simulink model "model_tmp_4p"  (R2015b)
settings: Solver=ode45  StartTime=0.0  StopTime=T_sim  FixedStep=dt  RelTol=1e-3
PreLoadFcn:
  | setup_tmp_4p;
InitFcn:
  | setup_tmp_4p;
StartFcn:
  | setup_tmp_4p;
values from neighbouring files (symbols this model uses):
  A_act = [-100 0 0 0 0 -100 0 0 0 0 -100 0 ... (16 elements, 4x4)]    [CD_spline.mat]    (also in CL_spline.mat; setup.m = -100*eye(4); setup_tmp_1p.m = -100*eye(4); setup_tmp_4p.m = -100*eye(4))
  A_init = [1.0386 0 12.9]    [CD_spline.mat]    (also in CL_spline.mat; setup_KiteModel_4points.m = Pc_init + d_n_r * w_k * w_rel * [-1;0;0])
  A_Kite = 7    [CD_spline.mat]    (also in CL_spline.mat; setup.m = 10.18; setup_tmp_1p.m = 10.18; setup_tmp_4p.m = 10.18)
  A_prd = [0 0 0 -640 0 0 0 0 0 0 -640 0 ... (36 elements, 6x6)]    [CD_spline.mat]    (also in CL_spline.mat; setup.m = 1000 * A_M_aug; setup_tmp_1p.m = 1000 * A_M_aug; setup_tmp_4p.m = 1000 * A_M_aug)
  A_ref = [0 0 0 -10000 0 0 0 0 0 0 -10000 0 ... (36 elements, 6x6)]    [CD_spline.mat]    (also in CL_spline.mat; setup.m = zeros(6); setup_tmp_1p.m = zeros(6); setup_tmp_4p.m = zeros(6))
  A_t_ref_cl = [0 0 0 -0.64 0 0 0 0 0 0 -0.64 0 ... (36 elements, 6x6)]    [CD_spline.mat]    (also in CL_spline.mat; setup.m = A_t_ref; setup_tmp_1p.m = A_t_ref; setup_tmp_4p.m = A_t_ref)
  alpha_0 = 10 * pi/180    (= 0.174532925199)    [setup_KiteModel_4points.m]
  alpha_d_max = 31 * pi/180    (= 0.541052068118)    [setup_KiteModel_4points.m]
  alpha_s_0 = 10 * pi/180    (= 0.174532925199)    [setup_KiteModel_4points.m]
  alpha_s_max = 20 * pi/180    (= 0.349065850399)    [setup_KiteModel_4points.m]
  ASideRel = 0    [CD_spline.mat]    (also in CL_spline.mat; setup.m; setup_tmp_1p.m; setup_tmp_4p.m = 0.306)
  B_act = [100 0 0 0 0 100 0 0 0 0 100 0 ... (16 elements, 4x4)]    [CD_spline.mat]    (also in CL_spline.mat; setup.m = 100*eye(4); setup_tmp_1p.m = 100*eye(4); setup_tmp_4p.m = 100*eye(4))
  B_init = [0 0 15.13]    [CD_spline.mat]    (also in CL_spline.mat; setup_KiteModel_4points.m = Pc_init + h_kite * [0;0;1;])
  B_ref = [0 0 0 10000 0 0 0 0 0 0 10000 0 ... (18 elements, 6x3)]    [CD_spline.mat]    (also in CL_spline.mat; setup.m = zeros(6,3); setup_tmp_1p.m = zeros(6,3); setup_tmp_4p.m = zeros(6,3))
  B_t_ref_cl = [0 0 0 0.64 0 0 0 0 0 0 0.64 0 ... (18 elements, 6x3)]    [CD_spline.mat]    (also in CL_spline.mat)
  Bpbl = [0 0 0 1 0 0 0 0 0 0 1 0 ... (18 elements, 6x3)]    [CD_spline.mat]    (also in CL_spline.mat; setup.m = [zeros(3); eye(3)]; setup_tmp_1p.m = [zeros(3); eye(3)]; setup_tmp_4p.m = [zeros(3); eye(3)])
  c0 = 614000    [CD_spline.mat]    (also in CL_spline.mat; setup.m; setup_tmp_1p.m; setup_tmp_4p.m)
  c_1_TR = 0.262    [setup_KiteModel_4points.m]
  C_A = [0 0.3 -1e-06 1 -0.3 0 1e-06 1 0 -0.3 -1e-06 1 ... (16 elements, 4x4)]    [CD_spline.mat]    (also in CL_spline.mat; setup.m = [0, -R, 0, R; setup_tmp_1p.m = [0, -R, 0, R; setup_tmp_4p.m = [0, -R, 0, R)
  C_A_inv = [0 -1.66666666667 -1.23358113847e-17 1.66666666667 1.66666666667 2.46716227694e-17 -1.66666666667 0 -250000 250000 -250000 250000 ... (16 elements, 4x4)]    [CD_spline.mat]    (also in CL_spline.mat; setup.m = C_A \eye(4); setup_tmp_1p.m = C_A \eye(4); setup_tmp_4p.m = C_A \eye(4))
  C_init = [0 2.5965 12.9]    [CD_spline.mat]    (also in CL_spline.mat; setup_KiteModel_4points.m = Pc_init + 0.5 * w_k * w_rel * [0;1;0])
  CD_spline_coefs = CD_spline.coefs    [setup_KiteModel_4points.m]
  CD_tether = 0.96    [CD_spline.mat]    (also in CL_spline.mat; setup.m; setup_tmp_1p.m; setup_tmp_4p.m)
  CL_spline_coefs = CL_spline.coefs    [setup_KiteModel_4points.m]
  d0 = 473    [CD_spline.mat]    (also in CL_spline.mat; setup.m; setup_tmp_1p.m; setup_tmp_4p.m)
  D_init = [0 -2.5965 12.9]    [CD_spline.mat]    (also in CL_spline.mat; setup_KiteModel_4points.m = Pc_init - 0.5 * w_k * w_rel * [0;1;0])
  d_tether = 0.004    [CD_spline.mat]    (also in CL_spline.mat; setup.m; setup_tmp_1p.m; setup_tmp_4p.m)
  delta_dead = 0.5    [CD_spline.mat]    (also in CL_spline.mat; setup.m; setup_tmp_1p.m; setup_tmp_4p.m)
  e_0 = 0.01    [CD_spline.mat]    (also in CL_spline.mat; setup.m; setup_tmp_1p.m; setup_tmp_4p.m)
  epsilon = 0.6    [CD_spline.mat]    (also in CL_spline.mat; setup.m; setup_tmp_1p.m; setup_tmp_4p.m)
  g = 9.81    [CD_spline.mat]    (also in CL_spline.mat; setup.m; setup_tmp_1p.m; setup_tmp_4p.m)
  g_vec = [0 0 9.81]    [CD_spline.mat]    (also in CL_spline.mat; setup.m = [0;0;9.81]; setup_tmp_1p.m = [0;0;9.81]; setup_tmp_4p.m = [0;0;9.81])
  Gamma_ad = 100    [CD_spline.mat]    (also in CL_spline.mat; setup.m = 100;100; setup_tmp_1p.m = 100;100; setup_tmp_4p.m = 100;100)
  Gamma_pred = 100    [CD_spline.mat]    (also in CL_spline.mat; setup.m; setup_tmp_1p.m; setup_tmp_4p.m)
  J = [0.018  0  0; 0  0.018  0; 0  0  0.009]    [CD_spline.mat]    (also in CL_spline.mat; setup.m = diag([Ixx, Iyy, Izz]); setup_tmp_1p.m = diag([Ixx, Iyy, Izz]); setup_tmp_4p.m = diag([Ixx, Iyy, Izz]))
  Jinv = [55.5555555556  0  0; 0  55.5555555556  0; 0  0  111.111111111]    [CD_spline.mat]    (also in CL_spline.mat; setup.m = J \ eye(3); setup_tmp_1p.m = J \ eye(3); setup_tmp_4p.m = J \ eye(3))
  K = 1 - ASideRel    [setup_KiteModel_4points.m]
  K_d_s = 1.5    [setup_KiteModel_4points.m]
  k_e_eta = 10000    [CD_spline.mat]    (also in CL_spline.mat; setup.m; setup_tmp_1p.m; setup_tmp_4p.m)
  k_e_eta_dot = 400    [CD_spline.mat]    (also in CL_spline.mat; setup.m; setup_tmp_1p.m; setup_tmp_4p.m)
  k_e_eta_I = 1    [CD_spline.mat]    (also in CL_spline.mat; setup.m; setup_tmp_1p.m; setup_tmp_4p.m)
  K_e_psi = 10    [setup_tmp_4p.m]
  K_i_t = [10  0  0; 0  10  0; 0  0  10]    [CD_spline.mat]    (also in CL_spline.mat; setup.m = 10*eye(3); setup_tmp_1p.m = 10*eye(3); setup_tmp_4p.m = 10*eye(3))
  K_v_t = [1.6  0  0; 0  1.6  0; 0  0  1.6]    [CD_spline.mat]    (also in CL_spline.mat; setup.m = 2*omega_0_trans*zeta_0_trans*eye(3); setup_tmp_1p.m = 2*omega_0_trans*zeta_0_trans*eye(3); setup_tmp_4p.m = 2*omega_0_trans*zeta_0_trans*eye(3))
  K_x_t = [0.64  0  0; 0  0.64  0; 0  0  0.64]    [CD_spline.mat]    (also in CL_spline.mat; setup.m = omega_0_trans^2*eye(3); setup_tmp_1p.m = omega_0_trans^2*eye(3); setup_tmp_4p.m = omega_0_trans^2*eye(3))
  l_s0 = 1    [CD_spline.mat]    (also in CL_spline.mat; setup.m = 1.42857142857; setup_tmp_1p.m = 1.42857142857; setup_tmp_4p.m = 2)
  l_s_BP = norm( B_init - p_B_UAV_init)    [setup_KiteModel_4points.m]
  l_s_PUav = norm( pos_UAV_init - p_B_UAV_init)    [setup_KiteModel_4points.m]
  ls_AB = norm( A_init -  B_init)    [setup_KiteModel_4points.m]
  ls_AC = norm( A_init -  C_init)    [setup_KiteModel_4points.m]
  ls_AD = norm( A_init -  D_init)    [setup_KiteModel_4points.m]
  ls_AKcu = norm( A_init -  P_kcu)    [setup_KiteModel_4points.m]
  ls_CB = norm( C_init -  B_init)    [setup_KiteModel_4points.m]
  ls_CD = norm( C_init -  D_init)    [setup_KiteModel_4points.m]
  ls_CKcu = norm( C_init - P_kcu)    [setup_KiteModel_4points.m]
  ls_DB = norm( D_init - B_init )    [setup_KiteModel_4points.m]
  ls_DKcu = norm( D_init - P_kcu)    [setup_KiteModel_4points.m]
  m_A = 3.29    [CD_spline.mat]    (also in CL_spline.mat; setup_KiteModel_4points.m = nose_mass_fraction * m_kite)
  m_B = 1.484    [CD_spline.mat]    (also in CL_spline.mat; setup_KiteModel_4points.m = 0.4 * (1-nose_mass_fraction)*m_kite)
  m_C = 1.113    [CD_spline.mat]    (also in CL_spline.mat; setup_KiteModel_4points.m = 0.3 * (1-nose_mass_fraction)*m_kite)
  m_D = 1.113    [CD_spline.mat]    (also in CL_spline.mat; setup_KiteModel_4points.m = 0.3 * (1-nose_mass_fraction)*m_kite)
  m_kcu = 8.4    [setup_tmp_4p.m]
  m_p = 0.013    [CD_spline.mat]    (also in CL_spline.mat; setup.m = 0.0185714285714; setup_tmp_1p.m = 0.0185714285714; setup_tmp_4p.m = 0.026)
  m_uav = 3    [CD_spline.mat]    (also in CL_spline.mat; setup.m; setup_tmp_1p.m; setup_tmp_4p.m)
  n_t_p = 7    [setup.m]    (also in setup_tmp_1p.m; setup_tmp_4p.m = 5)
  p_B_UAV_init = B_init + [0;0;l_s0]    [setup_KiteModel_4points.m]
  p_init_4p = zeros(3*n_t_p,1)    [setup.m]    (also in setup_tmp_4p.m)
  P_prd = [712.5 0 0 156.25 0 0 0 712.5 0 0 156.25 0 ... (36 elements, 6x6)]    [CD_spline.mat]    (also in CL_spline.mat; setup.m = 1000 * P_tref; setup_tmp_1p.m = 1000 * P_tref; setup_tmp_4p.m = 1000 * P_tref)
  P_tref = [0.7125 0 0 0.15625 0 0 0 0.7125 0 0 0.15625 0 ... (36 elements, 6x6)]    [CD_spline.mat]    (also in CL_spline.mat; setup.m = lyap(A_M_aug', Q); setup_tmp_1p.m = lyap(A_M_aug', Q); setup_tmp_4p.m = lyap(A_M_aug', Q))
  pos_UAV_init = p_B_UAV_init + [0;0;l_s0]    [setup_KiteModel_4points.m]
  rho_air = 1.225    [CD_spline.mat]    (also in CL_spline.mat; setup.m; setup_tmp_1p.m; setup_tmp_4p.m)
  rho_t = 0.013    [CD_spline.mat]    (also in CL_spline.mat; setup.m; setup_tmp_1p.m; setup_tmp_4p.m)
  sample_log = 0.01    [CD_spline.mat]    (also in CL_spline.mat; setup.m; setup_tmp_1p.m; setup_tmp_4p.m)
  T_launch = 40    [CD_spline.mat]    (also in CL_spline.mat; setup.m; setup_tmp_1p.m; setup_tmp_4p.m)
  Theta_max = 60    [CD_spline.mat]    (also in CL_spline.mat; setup.m; setup_tmp_1p.m; setup_tmp_4p.m)
  Thrust_Max = 80    [CD_spline.mat]    (also in CL_spline.mat; setup.m; setup_tmp_1p.m = 100; setup_tmp_4p.m = 1000000000)
  Tx = 10    [CD_spline.mat]    (also in CL_spline.mat; setup.m; setup_tmp_1p.m; setup_tmp_4p.m)
  Ty = 10    [CD_spline.mat]    (also in CL_spline.mat; setup.m; setup_tmp_1p.m; setup_tmp_4p.m)
  Tz = 10    [CD_spline.mat]    (also in CL_spline.mat; setup.m; setup_tmp_1p.m; setup_tmp_4p.m)
  u_d_0 = 0.213    [setup_KiteModel_4points.m]
  u_d_max = 0.47    [setup_KiteModel_4points.m]
  u_s_0 = 0    [setup_KiteModel_4points.m]
  v_w_vec = [1 1 1]    [CD_spline.mat]    (also in CL_spline.mat; setup.m = [1;0;0]; setup_tmp_1p.m = [1;0;0]; setup_tmp_4p.m = [0.01;0;0])
  x0num = 0    [CD_spline.mat]    (also in CL_spline.mat; polynomial_trajectory.m = double( solutions_x.x0 ))
  x1num = 0    [CD_spline.mat]    (also in CL_spline.mat; polynomial_trajectory.m = double( solutions_x.x1 ))
  x2num = 0    [CD_spline.mat]    (also in CL_spline.mat; polynomial_trajectory.m = double( solutions_x.x2 ))
  x3num = 0.05    [CD_spline.mat]    (also in CL_spline.mat; polynomial_trajectory.m = double( solutions_x.x3 ))
  x4num = -0.0075    [CD_spline.mat]    (also in CL_spline.mat; polynomial_trajectory.m = double( solutions_x.x4 ))
  x5num = 0.0003    [CD_spline.mat]    (also in CL_spline.mat; polynomial_trajectory.m = double( solutions_x.x5 ))
  x_drone_init = [0 0 10]    [CD_spline.mat]    (also in CL_spline.mat; setup.m = p_init(3*n-2:3*n); setup_KiteModel_4points.m = pos_UAV_init; setup_tmp_1p.m = p_init(3*n-2:3*n))
  xT = 5    [CD_spline.mat]    (also in CL_spline.mat; setup.m; setup_tmp_1p.m = 10; setup_tmp_4p.m = 10)
  y0num = 0    [CD_spline.mat]    (also in CL_spline.mat; polynomial_trajectory.m = double( solutions_y.y0 ))
  y1num = 0    [CD_spline.mat]    (also in CL_spline.mat; polynomial_trajectory.m = double( solutions_y.y1 ))
  y2num = 0    [CD_spline.mat]    (also in CL_spline.mat; polynomial_trajectory.m = double( solutions_y.y2 ))
  y3num = 0.1    [CD_spline.mat]    (also in CL_spline.mat; polynomial_trajectory.m = double( solutions_y.y3 ))
  y4num = -0.015    [CD_spline.mat]    (also in CL_spline.mat; polynomial_trajectory.m = double( solutions_y.y4 ))
  y5num = 0.0006    [CD_spline.mat]    (also in CL_spline.mat; polynomial_trajectory.m = double( solutions_y.y5 ))
  yT = 10    [CD_spline.mat]    (also in CL_spline.mat; setup.m; setup_tmp_1p.m = 0; setup_tmp_4p.m = 0)
  z0num = 10    [CD_spline.mat]    (also in CL_spline.mat; polynomial_trajectory.m = double( solutions_z.z0 ))
  z1num = 0    [CD_spline.mat]    (also in CL_spline.mat; polynomial_trajectory.m = double( solutions_z.z1 ))
  z2num = 0    [CD_spline.mat]    (also in CL_spline.mat; polynomial_trajectory.m = double( solutions_z.z2 ))
  z3num = 0.4    [CD_spline.mat]    (also in CL_spline.mat; polynomial_trajectory.m = double( solutions_z.z3 ))
  z4num = -0.06    [CD_spline.mat]    (also in CL_spline.mat; polynomial_trajectory.m = double( solutions_z.z4 ))
  z5num = 0.0024    [CD_spline.mat]    (also in CL_spline.mat; polynomial_trajectory.m = double( solutions_z.z5 ))
  zT = 50    [CD_spline.mat]    (also in CL_spline.mat; setup.m; setup_tmp_1p.m; setup_tmp_4p.m)
libraries: simulink x1
(part 2 of 3)

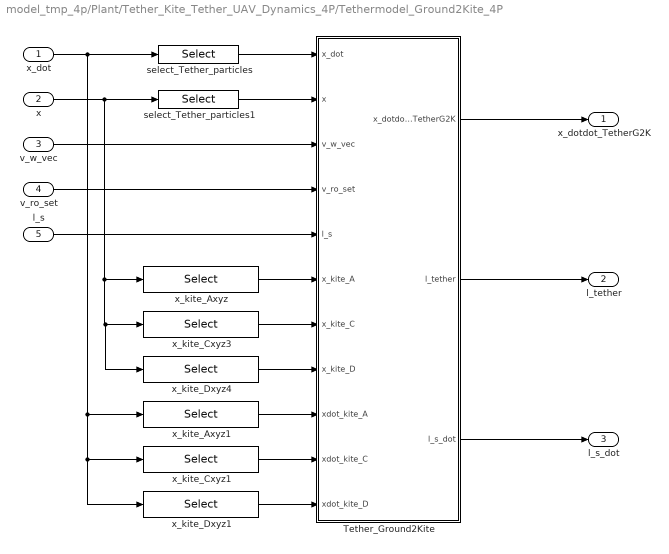
== system model_tmp_4p/Plant/Tether_Kite_Tether_UAV_Dynamics_4P/Tethermodel_Ground2Kite_4P ==
  x_dot : Inport
  x : Inport  Port=2
  v_w_vec : Inport  Port=3
  v_ro_set : Inport  Port=4
  l_s : Inport  Port=5
  Tether_Ground2Kite : MATLAB Function  TreatAsAtomicUnit=on
  select_Tether_particles : Selector  InputPortWidth=3*n_t_p+18  IndexOptions=Index vector (dialog)  Indices=[1 : 3*n_t_p]  OutputSizes=1
  select_Tether_particles1 : Selector  InputPortWidth=3*n_t_p+18  IndexOptions=Index vector (dialog)  Indices=[1 : 3*n_t_p]  OutputSizes=1
  x_kite_Axyz : Selector  InputPortWidth=3*n_t_p+18  IndexOptions=Index vector (dialog)  Indices=[3*n_t_p+1:3*n_t_p+3]  OutputSizes=1
  x_kite_Axyz1 : Selector  InputPortWidth=3*n_t_p+18  IndexOptions=Index vector (dialog)  Indices=[3*n_t_p+1:3*n_t_p+3]  OutputSizes=1
  x_kite_Cxyz1 : Selector  InputPortWidth=3*n_t_p+18  IndexOptions=Index vector (dialog)  Indices=[3*n_t_p+7:3*n_t_p+9]  OutputSizes=1
  x_kite_Cxyz3 : Selector  InputPortWidth=3*n_t_p+18  IndexOptions=Index vector (dialog)  Indices=[3*n_t_p+7:3*n_t_p+9]  OutputSizes=1
  x_kite_Dxyz1 : Selector  InputPortWidth=3*n_t_p+18  IndexOptions=Index vector (dialog)  Indices=[3*n_t_p+10:3*n_t_p+12]  OutputSizes=1
  x_kite_Dxyz4 : Selector  InputPortWidth=3*n_t_p+18  IndexOptions=Index vector (dialog)  Indices=[3*n_t_p+10:3*n_t_p+12]  OutputSizes=1
  x_dotdot_TetherG2K : Outport
  l_tether : Outport  Port=2
  l_s_dot : Outport  Port=3
  wires:
  v_w_vec/1 -> Tether_Ground2Kite/3(v_w_vec)
  x_dot/1 -> x_kite_Dxyz1/1, x_kite_Cxyz1/1, x_kite_Axyz1/1, select_Tether_particles/1
  x/1 -> x_kite_Dxyz4/1, x_kite_Cxyz3/1, x_kite_Axyz/1, select_Tether_particles1/1
  Tether_Ground2Kite/1(x_dotdot_TetherG2K) -> x_dotdot_TetherG2K/1
  Tether_Ground2Kite/2(l_tether) -> l_tether/1
  Tether_Ground2Kite/3(l_s_dot) -> l_s_dot/1
  l_s/1 -> Tether_Ground2Kite/5(l_s)
  v_ro_set/1 -> Tether_Ground2Kite/4(v_ro_set)
  select_Tether_particles/1 -> Tether_Ground2Kite/1(x_dot)
  select_Tether_particles1/1 -> Tether_Ground2Kite/2(x)
  x_kite_Axyz/1 -> Tether_Ground2Kite/6(x_kite_A)
  x_kite_Cxyz3/1 -> Tether_Ground2Kite/7(x_kite_C)
  x_kite_Dxyz4/1 -> Tether_Ground2Kite/8(x_kite_D)
  x_kite_Axyz1/1 -> Tether_Ground2Kite/9(xdot_kite_A)
  x_kite_Dxyz1/1 -> Tether_Ground2Kite/11(xdot_kite_D)
  x_kite_Cxyz1/1 -> Tether_Ground2Kite/10(xdot_kite_C)

== system model_tmp_4p/Plant/Tether_Kite_Tether_UAV_Dynamics_4P/Tethermodel_Kite2UAV ==
  x_p_dot : Inport
  launch_flag : Inport  Port=2
  x_p : Inport  Port=3
  v_w_vec : Inport  Port=4
  Tether_Kite2UAV : MATLAB Function  TreatAsAtomicUnit=on
  particle between uav and kite : Selector  InputPortWidth=3*n_t_p +18  IndexOptions=Index vector (dialog)  Indices=[3*n_t_p+13: 3*n_t_p+15]  OutputSizes=1
  particle between uav and kite1 : Selector  InputPortWidth=3*n_t_p +18  IndexOptions=Index vector (dialog)  Indices=[3*n_t_p+13: 3*n_t_p+15]  OutputSizes=1
  uav : Selector  InputPortWidth=3*n_t_p +18  IndexOptions=Index vector (dialog)  Indices=[3*n_t_p + 16: 3*n_t_p + 18]  OutputSizes=1
  x_kite_B : Selector  InputPortWidth=3*n_t_p +18  IndexOptions=Index vector (dialog)  Indices=[3*n_t_p + 4: 3*n_t_p + 6]  OutputSizes=1
  x_kite_B1 : Selector  InputPortWidth=3*n_t_p +18  IndexOptions=Index vector (dialog)  Indices=[3*n_t_p + 4: 3*n_t_p + 6]  OutputSizes=1
  x_kite_B5 : Selector  InputPortWidth=3*n_t_p +18  IndexOptions=Index vector (dialog)  Indices=[3*n_t_p + 16: 3*n_t_p + 18]  OutputSizes=1
  x_dotdot_p : Outport
  wires:
  Tether_Kite2UAV/1(x_dotdot_p) -> x_dotdot_p/1
  launch_flag/1 -> Tether_Kite2UAV/1(launch_flag)
  uav/1 -> Tether_Kite2UAV/2(xp_above)
  x_kite_B1/1 -> Tether_Kite2UAV/7(xp_dot_below)
  x_p_dot/1 -> particle between uav and kite1/1, x_kite_B1/1, x_kite_B5/1
  particle between uav and kite/1 -> Tether_Kite2UAV/3(xp)
  x_kite_B5/1 -> Tether_Kite2UAV/5(xp_dot_above)
  x_p/1 -> uav/1, particle between uav and kite/1, x_kite_B/1
  x_kite_B/1 -> Tether_Kite2UAV/4(xp_below)
  v_w_vec/1 -> Tether_Kite2UAV/8(v_w_vec)
  particle between uav and kite1/1 -> Tether_Kite2UAV/6(xp_dot)

== system model_tmp_4p/Plant/Tether_Kite_Tether_UAV_Dynamics_4P/UAV_Model ==
  x_p_dot : Inport
  x_p : Inport  Port=2
  u_M : Inport  Port=3
  u_Thrust_I : Inport  Port=4
  eta : Inport  Port=5
  omega : Inport  Port=6
  Kite1 : Selector  InputPortWidth=3*n_t_p + 18  IndexOptions=Index vector (dialog)  Indices=[3*n_t_p + 16:3*n_t_p + 18]  OutputSizes=1
  Kite2 : Selector  InputPortWidth=3*n_t_p + 18  IndexOptions=Index vector (dialog)  Indices=[3*n_t_p + 16:3*n_t_p + 18]  OutputSizes=1
  Kite3 : Selector  InputPortWidth=3*n_t_p + 18  IndexOptions=Index vector (dialog)  Indices=[3*n_t_p + 13:3*n_t_p + 15]  OutputSizes=1
  Kite4 : Selector  InputPortWidth=3*n_t_p + 18  IndexOptions=Index vector (dialog)  Indices=[3*n_t_p + 13:3*n_t_p + 15]  OutputSizes=1
  Rotate thrust vector according to attitude : MATLAB Function  TreatAsAtomicUnit=on
  To Workspace4 : ToWorkspace  VariableName=F_T_b  SaveFormat=Timeseries  SampleTime=sample_log
  UAV_Dynamics : MATLAB Function  TreatAsAtomicUnit=on
  x_dotdot_uav : Outport
  omega_dot : Outport  Port=2
  eta_dot : Outport  Port=3
  tag scope: disturbance=global
  wires:
  Rotate thrust vector according to attitude/1(u_Thrust_B) -> To Workspace4/1, UAV_Dynamics/1(Thrust)
  UAV_Dynamics/1(x_dotdot_uav_trans) -> x_dotdot_uav/1
  Kite1/1 -> UAV_Dynamics/2(x_UAV)
  Kite4/1 -> UAV_Dynamics/5(x_dot_belowUAV)
  Kite2/1 -> UAV_Dynamics/4(x_dot_UAV)
  x_p_dot/1 -> Kite4/1, Kite2/1
  x_p/1 -> Kite3/1, Kite1/1
  UAV_Dynamics/4(disturbance) -> [disturbance]
  UAV_Dynamics/2(omega_dot) -> omega_dot/1
  UAV_Dynamics/3(eta_dot) -> eta_dot/1
  u_M/1 -> UAV_Dynamics/7(u_M)
  eta/1 -> Rotate thrust vector according to attitude/2(eta), UAV_Dynamics/8(eta)
  omega/1 -> UAV_Dynamics/6(omega)
  u_Thrust_I/1 -> Rotate thrust vector according to attitude/1(u_Thrust_I)
  Kite3/1 -> UAV_Dynamics/3(x_below_UAV)

== system model_tmp_4p/Controller/Outer_Loop_Position/Adaptive_Augmentation/Proj(Theta_hat, GammaY)_1column ==
  note: Ref.: Lavretsky, Robust and Adaptive Control, p. 329
      | Lecure Notes Nonlinear and Adaptive Control, TU Munich, FSD, SS2014, Robustness Modifications
  Theta_hat : Inport
  Theta_dot : Inport  Port=2
  Mux : Mux  Inputs=3
  Proj(Theta,Theta_dot) : MATLAB Function  TreatAsAtomicUnit=on
  Reshape1 : Reshape  OutputDimensionality=Row vector (2-D)
  Reshape2 : Reshape  OutputDimensionality=Row vector (2-D)
  To Workspace1 : ToWorkspace  VariableName=proj_flat  SaveFormat=Timeseries  SampleTime=sample_log
      settings: Save2DSignal=2-D array (concatenate along first dimension)
  To Workspace2 : ToWorkspace  VariableName=Theta_dot_save  SampleTime=sample_log
      settings: Save2DSignal=2-D array (concatenate along first dimension)
  To Workspace3 : ToWorkspace  VariableName=orthogonal_part  SampleTime=sample_log
      settings: Save2DSignal=2-D array (concatenate along first dimension)
  calculate_f : MATLAB Function  TreatAsAtomicUnit=on
  calculate_gradf : MATLAB Function  TreatAsAtomicUnit=on
  max_allowable_bound : Constant  Value=Theta_max
  projection_tolerance : Constant  Value=epsilon
  Theta_hat_dot : Outport
  wires:
  Proj(Theta,Theta_dot)/2(Theta_hat_dot_) -> Reshape1/1, Theta_hat_dot/1
  Proj(Theta,Theta_dot)/1(flag) -> Mux/2
  Proj(Theta,Theta_dot)/3(direction) -> Mux/3
  Mux/1 -> To Workspace1/1
  calculate_gradf/1(gradf) -> Proj(Theta,Theta_dot)/2(gradf)
  Theta_hat/1 -> calculate_gradf/1(theta_hat), calculate_f/1(theta_hat)
  projection_tolerance/1 -> calculate_f/3(epsilon), calculate_gradf/3(epsilon)
  max_allowable_bound/1 -> calculate_f/2(Theta_max), calculate_gradf/2(Theta_max)
  Theta_dot/1 -> Proj(Theta,Theta_dot)/3(Theta_dot)
  calculate_f/1(f) -> Mux/1, Proj(Theta,Theta_dot)/1(f)
  Reshape1/1 -> To Workspace2/1
  Proj(Theta,Theta_dot)/4(orthogonal_part) -> Reshape2/1
  Reshape2/1 -> To Workspace3/1

== system model_tmp_4p/Controller/Outer_Loop_Position/Adaptive_Augmentation/Proj(Theta_hat, GammaY)_multicolumns ==
  note: Ref.: Lavretsky, Robust and Adaptive Control, p. 329
      | Lecure Notes Nonlinear and Adaptive Control, TU Munich, FSD, SS2014, Robustness Modifications
  Theta_hat : Inport
  Theta_dot : Inport  Port=2
  MATLAB Function : MATLAB Function  TreatAsAtomicUnit=on
  Matrix Concatenate : Concatenate  NumInputs=3  Mode=Multidimensional array
  Projection_Input_1 : Subsystem
  Projection_Input_2 : Subsystem
  Projection_Input_3 : Subsystem
  Theta_hat_dot : Outport
  wires:
  Theta_hat/1 -> MATLAB Function/1(Theta_hat)
  Theta_dot/1 -> MATLAB Function/2(Theta_hat_dot)
  Projection_Input_1/1(Out1) -> Matrix Concatenate/1
  MATLAB Function/1(Theta_hat_1) -> Projection_Input_1/1(In1)
  MATLAB Function/2(Theta_hat_dot_1) -> Projection_Input_1/2(In2)
  MATLAB Function/3(Theta_hat_2) -> Projection_Input_2/1(In1)
  MATLAB Function/4(Theta_hat_dot_2) -> Projection_Input_2/2(In2)
  MATLAB Function/6(Theta_hat_dot_3) -> Projection_Input_3/2(In2)
  MATLAB Function/5(Theta_hat_3) -> Projection_Input_3/1(In1)
  Projection_Input_2/1(Out1) -> Matrix Concatenate/2
  Projection_Input_3/1(Out1) -> Matrix Concatenate/3
  Matrix Concatenate/1 -> Theta_hat_dot/1

== system model_tmp_4p/Controller/Outer_Loop_Position/Adaptive_Augmentation/Smooth_Deadzone_MRAC ==
  note: Ref.: Lavretsky, Robust and Adaptive Control, p. 319
  e : Inport
  Dead_Zone_Mod1 : Constant  Value=delta_dead
  Dead_Zone_Mod2 : Constant  Value=e_0
  Dot Product : DotProduct  InputSameDT=on  OutDataTypeStr=Inherit: Inherit via internal rule
  Mux : Mux  Inputs=2
  Sqrt : Sqrt  SaturateOnIntegerOverflow=on
  To Workspace8 : ToWorkspace  VariableName=e_ref_mu  SaveFormat=Timeseries  SampleTime=sample_log
      settings: Save2DSignal=2-D array (concatenate along first dimension)
  smooth_deadzone : MATLAB Function  TreatAsAtomicUnit=on
  mu_dead : Outport
  wires:
  e/1 -> Dot Product/1, Dot Product/2
  Dead_Zone_Mod1/1 -> smooth_deadzone/2(delta_dead)
  Dead_Zone_Mod2/1 -> smooth_deadzone/3(e_0)
  Dot Product/1 -> Sqrt/1
  Sqrt/1 -> Mux/1, smooth_deadzone/1(e_norm)
  smooth_deadzone/1(mu_dead) -> Mux/2, mu_dead/1
  Mux/1 -> To Workspace8/1

== system model_tmp_4p/Controller/Outer_Loop_Position/Adaptive_Augmentation/Smooth_Deadzone_PMRAC ==
  note: Ref.: Lavretsky, Robust and Adaptive Control, p. 319
  e : Inport
  Dead_Zone_Mod1 : Constant  Value=delta_dead
  Dead_Zone_Mod2 : Constant  Value=e_0
  Dot Product : DotProduct  InputSameDT=on  OutDataTypeStr=Inherit: Inherit via internal rule
  Mux1 : Mux  Inputs=2
  Sqrt : Sqrt  SaturateOnIntegerOverflow=on
  To Workspace1 : ToWorkspace  VariableName=e_pref_mu  SaveFormat=Timeseries  SampleTime=sample_log
      settings: Save2DSignal=2-D array (concatenate along first dimension)
  smooth_deadzone : MATLAB Function  TreatAsAtomicUnit=on
  mu_dead : Outport
  wires:
  Dot Product/1 -> Sqrt/1
  Dead_Zone_Mod2/1 -> smooth_deadzone/3(e_0)
  Dead_Zone_Mod1/1 -> smooth_deadzone/2(delta_dead)
  e/1 -> Dot Product/2, Dot Product/1
  Sqrt/1 -> Mux1/1, smooth_deadzone/1(e_norm)
  smooth_deadzone/1(mu_dead) -> Mux1/2, mu_dead/1
  Mux1/1 -> To Workspace1/1

== system model_tmp_4p/Plant/Tether_Kite_Tether_UAV_Dynamics_4P/First_order_lag_Actuator/Actuator ==
  Propeller_RPMs_cmd : Inport
  Add : Sum  Inputs=+-
  Gain : Gain  Gain=B_act  Multiplication=Matrix(K*u)
  Gain1 : Gain  Gain=A_act  Multiplication=Matrix(K*u)
  Integrator Limited1 : Integrator  InitialCondition=zeros(4,1)  LimitOutput=on  UpperSaturationLimit=Thrust_Max  LowerSaturationLimit=-Thrust_Max
  Output_Actuator : Gain  Gain=C_A  Multiplication=Matrix(K*u)
  Reaction_Deficit_Actuators : Scope
  Sum : Sum  Inputs=|++
  To Workspace1 : ToWorkspace  VariableName=prop_thrust_cmd  SaveFormat=Timeseries  SampleTime=sample_log
  To Workspace2 : ToWorkspace  VariableName=prop_thrust_real  SaveFormat=Timeseries  SampleTime=sample_log
  Thrust_Moments : Outport
  wires:
  Output_Actuator/1 -> Thrust_Moments/1
  Gain/1 -> Sum/1
  Gain1/1 -> Sum/2
  Sum/1 -> Integrator Limited1/1
  Propeller_RPMs_cmd/1 -> Add/1, To Workspace1/1, Gain/1
  Add/1 -> Reaction_Deficit_Actuators/1
  Integrator Limited1/1 -> Add/2, To Workspace2/1, Gain1/1, Output_Actuator/1

== system model_tmp_4p/Controller/Outer_Loop_Position/Adaptive_Augmentation/Proj(Theta_hat, GammaY)_multicolumns/Projection_Input_1 ==
  In1 : Inport
  In2 : Inport  Port=2
  Proj(Theta,Theta_dot) : MATLAB Function  TreatAsAtomicUnit=on
  calculate_f : MATLAB Function  TreatAsAtomicUnit=on
  calculate_gradf : MATLAB Function  TreatAsAtomicUnit=on
  max_allowable_bound : Constant  Value=Theta_max
  projection_tolerance : Constant  Value=epsilon
  Out1 : Outport
  wires:
  calculate_f/1(f) -> Proj(Theta,Theta_dot)/1(f)
  In2/1 -> Proj(Theta,Theta_dot)/3(Theta_dot)
  max_allowable_bound/1 -> calculate_f/2(Theta_max), calculate_gradf/2(Theta_max)
  projection_tolerance/1 -> calculate_f/3(epsilon), calculate_gradf/3(epsilon)
  In1/1 -> calculate_gradf/1(theta_hat), calculate_f/1(theta_hat)
  calculate_gradf/1(gradf) -> Proj(Theta,Theta_dot)/2(gradf)
  Proj(Theta,Theta_dot)/1(Theta_hat_dot_) -> Out1/1

== system model_tmp_4p/Controller/Outer_Loop_Position/Adaptive_Augmentation/Proj(Theta_hat, GammaY)_multicolumns/Projection_Input_2 ==
  In1 : Inport
  In2 : Inport  Port=2
  Proj(Theta,Theta_dot) : MATLAB Function  TreatAsAtomicUnit=on
  calculate_f : MATLAB Function  TreatAsAtomicUnit=on
  calculate_gradf : MATLAB Function  TreatAsAtomicUnit=on
  max_allowable_bound : Constant  Value=Theta_max
  projection_tolerance : Constant  Value=epsilon
  Out1 : Outport
  wires:
  calculate_f/1(f) -> Proj(Theta,Theta_dot)/1(f)
  In2/1 -> Proj(Theta,Theta_dot)/3(Theta_dot)
  max_allowable_bound/1 -> calculate_f/2(Theta_max), calculate_gradf/2(Theta_max)
  projection_tolerance/1 -> calculate_f/3(epsilon), calculate_gradf/3(epsilon)
  In1/1 -> calculate_gradf/1(theta_hat), calculate_f/1(theta_hat)
  calculate_gradf/1(gradf) -> Proj(Theta,Theta_dot)/2(gradf)
  Proj(Theta,Theta_dot)/1(Theta_hat_dot_) -> Out1/1

== system model_tmp_4p/Controller/Outer_Loop_Position/Adaptive_Augmentation/Proj(Theta_hat, GammaY)_multicolumns/Projection_Input_3 ==
  In1 : Inport
  In2 : Inport  Port=2
  Mux : Mux  Inputs=3
  Proj(Theta,Theta_dot) : MATLAB Function  TreatAsAtomicUnit=on
  Scope : Scope
  Scope1 : Scope
  To Workspace1 : ToWorkspace  VariableName=proj_flat  SaveFormat=Timeseries  SampleTime=sample_log
      settings: Save2DSignal=2-D array (concatenate along first dimension)
  calculate_f : MATLAB Function  TreatAsAtomicUnit=on
  calculate_gradf : MATLAB Function  TreatAsAtomicUnit=on
  max_allowable_bound : Constant  Value=Theta_max
  projection_tolerance : Constant  Value=epsilon
  Out1 : Outport
  wires:
  calculate_f/1(f) -> Mux/1, Proj(Theta,Theta_dot)/1(f)
  In2/1 -> Proj(Theta,Theta_dot)/3(Theta_dot)
  max_allowable_bound/1 -> calculate_f/2(Theta_max), calculate_gradf/2(Theta_max)
  projection_tolerance/1 -> calculate_f/3(epsilon), calculate_gradf/3(epsilon)
  In1/1 -> calculate_gradf/1(theta_hat), calculate_f/1(theta_hat)
  calculate_gradf/1(gradf) -> Proj(Theta,Theta_dot)/2(gradf)
  Proj(Theta,Theta_dot)/2(Theta_hat_dot_) -> Out1/1
  Mux/1 -> To Workspace1/1
  Proj(Theta,Theta_dot)/3(direction) -> Scope/1, Mux/3
  Proj(Theta,Theta_dot)/1(flag) -> Scope1/1, Mux/2

== matlab function model_tmp_4p/Controller/Inner_Loop_Attitude/Plant_Inversion_RD2/Plant_Inversion ==
  data: omega input; u_NDI output; eta input; eta_dot input; J input; nu_tot input
function u_NDI = fcn(omega, eta, eta_dot, J, nu_tot)
%#codegen
p = omega(1); 
q = omega(2); 
r = omega(3); 
Ix = J(1,1); 
Iy = J(2,2); 
Iz = J(3,3); 


cross_coupling = [ Iy*q*r - Iz*q*r
 Iz*p*r - Ix*p*r;
 Ix*p*q - Iy*p*q];

% T_inv = [1, sin(eta(1)) * tan(eta(2)), cos(eta(1)) * tan(eta(2)) ; 
% 0, cos(eta(1)), -sin(eta(1)); 
% 0, sin(eta(1))/cos(eta(2)), cos(eta(1))/cos(eta(2))] \ eye(3); 

T_inv = [1, 0, -sin(eta(2));
         0, cos(eta(1)), sin(eta(1))*cos(eta(2));
         0, -sin(eta(1)), cos(eta(1))*cos(eta(2))];
     
T_dot = eta_dot(1) * [0, cos(eta(1)) * tan(eta(2)), -sin(eta(1))*tan(eta(2)); 
                      0, -sin(eta(1)), -cos(eta(1));
                      0, cos(eta(1))/cos(eta(2)), -sin(eta(1))/cos(eta(2))]+...
        eta_dot(2) * [0, sin(eta(1))/cos(eta(2))^2, cos(eta(1))/cos(eta(2))^2; 
                       0, 0, 0; 
                       0, sin(eta(1))*sin(eta(2))/cos(eta(2))^2, cos(eta(1))*sin(eta(2))/cos(eta(2))^2];
                          
u_NDI = -cross_coupling + J * T_inv * ( -T_dot * omega + nu_tot);

== matlab function model_tmp_4p/Flight_Path_Planner/Reference_Dynamic_x1 ==
  data: t input; y_ref output; y0num parameter; y1num parameter; y2num parameter; y3num parameter; y4num parameter; y5num parameter; yT parameter; Ty parameter
function y_ref = fcn(t,y0num, y1num, y2num, y3num, y4num, y5num, yT,Ty )

if t >= Ty
    y_ref = yT;
else
    y_ref = y5num * t^5 + y4num * t^4 + y3num * t^3 + y2num * t^2 + y1num * t + y0num;
end

== matlab function model_tmp_4p/Flight_Path_Planner/Reference_Dynamic_x3 ==
  data: t input; x_ref output; x0num parameter; x1num parameter; x2num parameter; x3num parameter; x4num parameter; x5num parameter; Tx parameter; xT parameter
function x_ref = fcn(t,x0num, x1num, x2num, x3num, x4num, x5num, Tx,xT )

if t >= Tx
    x_ref = xT;
else
    x_ref = x5num * t^5 + x4num * t^4 + x3num * t^3 + x2num * t^2 + x1num * t + x0num;
end

== matlab function model_tmp_4p/Controller/Kite_Controller/Reference_Model_TurnrateLaw/Psi_reference_model ==
  data: Psi_ref_dot output; Psi_cmd input; a_TR_ref parameter; Psi_ref input
function Psi_ref_dot = fcn(Psi_cmd,a_TR_ref, Psi_ref)
%#codegen
Psi_ref_dot = -a_TR_ref * Psi_ref + a_TR_ref * Psi_cmd;

== matlab function model_tmp_4p/Controller/Inner_Loop_Attitude/estimate_eta_dot ==
  data: omega input; eta input; eta_dot output
function eta_dot  = fcn( omega, eta)
%#codegen

eta_dot = [1, sin(eta(1)) * tan(eta(2)), cos(eta(1)) * tan(eta(2)) ; 
0, cos(eta(1)), -sin(eta(1)); 
0, sin(eta(1))/cos(eta(2)), cos(eta(1))/cos(eta(2))] * omega;

== matlab function model_tmp_4p/Flight_Path_Planner/Reference_Dynamic_x2 ==
  data: t input; z_ref output; z0num parameter; z1num parameter; z2num parameter; z3num parameter; z4num parameter; z5num parameter; Tz parameter; zT parameter
function z_ref = fcn(t,z0num, z1num, z2num, z3num, z4num, z5num,Tz, zT)

if t >= Tz
    z_ref = zT;
else
    z_ref = z5num * t^5 + z4num * t^4 + z3num * t^3 + z2num * t^2 + z1num * t + z0num;
end

== matlab function model_tmp_4p/Controller/Outer_Loop_Position/Adaptive_Augmentation/Smooth_Deadzone_PMRAC/smooth_deadzone ==
  data: e_norm input; mu_dead output; delta_dead input; e_0 input
function mu_dead = fcn(e_norm, delta_dead, e_0)
%#codegen

mu_dead = max( 0, min( 1, (e_norm - delta_dead*e_0)/...
                          ( (1-delta_dead) * e_0) ) );

== matlab function model_tmp_4p/Controller/Kite_Controller/TRL_Inversion ==
  data: K_d_s parameter; u_NDI output; c_1_TR parameter; v_a input; u_d_0 parameter; u_d_max parameter; u_s_0 parameter; nu_tot input; u_d input
function u_NDI = fcn(K_d_s, c_1_TR, v_a, u_d_0, u_d_max, u_s_0, nu_tot, u_d)
%#codegen
v_a = sign(v_a) * max( abs(v_a), 0.1);
u_NDI = nu_tot/c_1_TR/v_a * ( 1 + K_d_s * ( u_d - u_d_0 )/(u_d_max - u_d_0) ) + u_s_0;

== matlab function model_tmp_4p/Controller/Outer_Loop_Position/Predictor_Model_Translational_Dynamics/Reference_Model_Position ==
  data: A_prd input; A_ref input; x_prd_dotdot output; B_ref input; x_cmd input; x_p input; x_prd input
function x_prd_dotdot  = fcn(A_prd,A_ref,B_ref, x_cmd,x_p,x_prd)

    x_prd_dotdot = A_prd * (x_prd - x_p) + A_ref * x_p + B_ref * x_cmd;

== matlab function model_tmp_4p/Controller/Outer_Loop_Position/Reference_Model_Translational_Dynamics/Reference_Model_Position ==
  data: A_t_ref_cl input; x_ref_dotdot output; B_t_ref input; x_cmd input; x_ref input
function x_ref_dotdot  = fcn(A_t_ref_cl,B_t_ref, x_cmd,x_ref)

    x_ref_dotdot = A_t_ref_cl * x_ref + B_t_ref * x_cmd;

== matlab function model_tmp_4p/Controller/Outer_Loop_Position/Adaptive_Augmentation/Proj(Theta_hat, GammaY)_multicolumns/MATLAB Function ==
  data: Theta_hat input; Theta_hat_1 output; Theta_hat_dot_1 output; Theta_hat_dot input; Theta_hat_2 output; Theta_hat_dot_2 output; Theta_hat_3 output; Theta_hat_dot_3 output
function [Theta_hat_1,Theta_hat_dot_1, Theta_hat_2, Theta_hat_dot_2,...
            Theta_hat_3, Theta_hat_dot_3] = fcn(Theta_hat, Theta_hat_dot)
%#codegen
Theta_hat_1 = Theta_hat(1,:);
Theta_hat_2 = Theta_hat(2,:);
Theta_hat_3 = Theta_hat(3,:);

Theta_hat_dot_1 = Theta_hat_dot(1,:); 
Theta_hat_dot_2 = Theta_hat_dot(2,:);
Theta_hat_dot_3 = Theta_hat_dot(3,:);

== matlab function model_tmp_4p/Controller/Outer_Loop_Position/Adaptive_Augmentation/Proj(Theta_hat, GammaY)_multicolumns/Projection_Input_1/Proj(Theta,Theta_dot) ==
  data: f input; gradf input; Theta_dot input; Theta_hat_dot_ output
function  Theta_hat_dot_ = fcn(f, gradf, Theta_dot )
%#codegen


if ( f > 0 && gradf*Theta_dot' > 0 )
    Theta_hat_dot_ = Theta_dot - f * ( (gradf'*gradf) / (gradf*gradf') * Theta_dot' )'   ;
else
    Theta_hat_dot_ =  Theta_dot;
end

== matlab function model_tmp_4p/Controller/Outer_Loop_Position/Total_Thrust ==
  data: T_ref input; T_tot output
function T_tot  = fcn(T_ref)

%T_z = [0;0;norm(T_ref)];
T_tot = norm(T_ref);

== matlab function model_tmp_4p/Controller/Outer_Loop_Position/Adaptive_Augmentation/Proj(Theta_hat, GammaY)_multicolumns/Projection_Input_1/calculate_f ==
  data: theta_hat input; f output; Theta_max input; epsilon input
function f   = fcn(theta_hat,Theta_max, epsilon )
%#codegen
f = ( (1+epsilon)*norm(theta_hat)^2 - (Theta_max)^2 ) / (epsilon*(Theta_max)^2);

== matlab function model_tmp_4p/Controller/Outer_Loop_Position/Adaptive_Augmentation/Proj(Theta_hat, GammaY)_multicolumns/Projection_Input_1/calculate_gradf ==
  data: theta_hat input; gradf output; Theta_max input; epsilon input
function gradf = fcn(theta_hat,Theta_max, epsilon )
%#codegen
gradf = ( 2*(1+epsilon) ) / (epsilon*(Theta_max)^2) * theta_hat ;

== matlab function model_tmp_4p/Controller/Pseudo_Control_Hedging/Rotate thrust vector according to attitude ==
  data: u_Thrust_I input; eta input; u_Thrust_B output
function u_Thrust_B   = thrust_Bz_direction(  u_Thrust_I, eta) 

phi = eta(1); 
theta = eta(2); 
psi = eta(3); 

% Rotate thrust vector such that it is perpendicular to the "rotor blades"
u_Thrust_B = [cos(psi)*cos(theta), sin(psi)*cos(theta), -sin(theta); 
            cos(psi)*sin(theta)*sin(phi)-sin(psi)*cos(phi), sin(psi)*sin(theta)*sin(phi)+cos(psi)*cos(phi), cos(theta)*sin(phi); 
            cos(psi)*sin(theta)*cos(phi)+sin(psi)*sin(phi), sin(psi)*sin(theta)*cos(phi)-cos(psi)*sin(phi), cos(theta)*cos(phi)] *...
            [0;0;u_Thrust_I];

== matlab function model_tmp_4p/Controller/Pseudo_Control_Hedging/Plant_Inversion_RD2_backwards/Plant_Inversion ==
  data: omega input; nu_tot_rot_hat output; eta input; eta_dot input; J parameter; Jinv parameter; M_hat input
function nu_tot_rot_hat = fcn(omega, eta, eta_dot,J, Jinv, M_hat)
%#codegen
p = omega(1); 
q = omega(2); 
r = omega(3); 
Ix = J(1,1); 
Iy = J(2,2); 
Iz = J(3,3); 


cross_coupling = [ Iy*q*r - Iz*q*r
 Iz*p*r - Ix*p*r;
 Ix*p*q - Iy*p*q];

% T_inv = [1, sin(eta(1)) * tan(eta(2)), cos(eta(1)) * tan(eta(2)) ; 
% 0, cos(eta(1)), -sin(eta(1)); 
% 0, sin(eta(1))/cos(eta(2)), cos(eta(1))/cos(eta(2))] \ eye(3); 

T = [1, sin(eta(1)) * tan(eta(2)), cos(eta(1)) * tan(eta(2)) ; 
0, cos(eta(1)), -sin(eta(1)); 
0, sin(eta(1))/cos(eta(2)), cos(eta(1))/cos(eta(2))];

T_dot = eta_dot(1) * [0, cos(eta(1)) * tan(eta(2)), -sin(eta(1))*tan(eta(2)); 
                      0, -sin(eta(1)), -cos(eta(1));
                      0, cos(eta(1))/cos(eta(2)), -sin(eta(1))/cos(eta(2))]+...
        eta_dot(2) * [0, sin(eta(1))/cos(eta(2))^2, cos(eta(1))/cos(eta(2))^2; 
                       0, 0, 0; 
                       0, sin(eta(1))*sin(eta(2))/cos(eta(2))^2, cos(eta(1))*sin(eta(2))/cos(eta(2))^2];
                          
%u_NDI = -cross_coupling + J * T_inv * ( -T_dot * omega + nu_tot); 

nu_tot_rot_hat = T * Jinv * ( M_hat + cross_coupling ) + T_dot *omega;

== matlab function model_tmp_4p/Controller/Pseudo_Control_Hedging/Plant_Inversion_RD2_backwards/estimate_eta_dot ==
  data: omega input; eta input; eta_dot output
function eta_dot  = fcn( omega, eta)
%#codegen

eta_dot = [1, sin(eta(1)) * tan(eta(2)), cos(eta(1)) * tan(eta(2)) ; 
0, cos(eta(1)), -sin(eta(1)); 
0, sin(eta(1))/cos(eta(2)), cos(eta(1))/cos(eta(2))] * omega;

== matlab function model_tmp_4p/Controller/Outer_Loop_Position/Adaptive_Augmentation/Smooth_Deadzone_MRAC/smooth_deadzone ==
  data: e_norm input; mu_dead output; delta_dead input; e_0 input
function mu_dead = fcn(e_norm, delta_dead, e_0)
%#codegen

mu_dead = max( 0, min( 1, (e_norm - delta_dead*e_0)/...
                          ( (1-delta_dead) * e_0) ) );

== matlab function model_tmp_4p/Controller/Outer_Loop_Position/Calc_Ref_Attitude ==
  data: T_ref input; Eta_Cmd output; eta input
function Eta_Cmd  = fcn(T_ref, eta)
%#codegen
psi = eta(3); 
theta = eta(2); 
phi = eta(1); 

psi_c = 0;

T = norm( T_ref ); 

phi_c = -asin( 1/T * (T_ref(1) * sin(psi_c) - T_ref(2) * cos(psi_c)) ); 
theta_c = -atan( 1/T_ref(3) * (T_ref(1) * cos(psi_c) + T_ref(2) * sin(psi_c))); 

Eta_Cmd = [phi_c;theta_c; 0];

== matlab function model_tmp_4p/Plant/Tether_Kite_Tether_UAV_Dynamics_4P/Kite_Model_4p/Kite_Model_4p ==
  data: x_dotdot_kite output; v_w_vec input; u_s input; u_d input; ASideRel parameter; alpha_0 parameter; alpha_s_0 parameter; u_s_0 parameter; alpha_s_max parameter; alpha_d_max parameter; u_d_max parameter; u_d_0 parameter; K_d_s parameter; x_kite_A input; x_kite_B input; x_kite_C input; x_kite_D input; x_kite_kcu input; x_above_kite input; xdot_kite_A input; xdot_kite_B input; xdot_kite_C input; xdot_kite_D input; xdot_kite_kcu input; xdot_above_kite input; CL_spline_coefs parameter; CD_spline_coefs parameter; rho_air parameter; A_Kite parameter; K parameter; g_vec parameter; m_A parameter; m_B parameter; m_C parameter; m_D parameter; d0 parameter; c0 parameter; ls_AC parameter; ls_AB parameter; ls_AKcu parameter; ls_AD parameter; ls_CB parameter; ls_CD parameter; ls_CKcu parameter; ls_DKcu parameter; ls_DB parameter; l_s_BP parameter; Psi_dot output; c_1_TR parameter
%% 4 Point kite implementation

function [x_dotdot_kite, Psi_dot]  = fcn( v_w_vec, u_s,u_d, ASideRel,alpha_0, alpha_s_0,u_s_0,alpha_s_max,...
    alpha_d_max, u_d_max, u_d_0, K_d_s, x_kite_A, x_kite_B, x_kite_C, x_kite_D, x_kite_kcu,...
    x_above_kite, xdot_kite_A, xdot_kite_B, xdot_kite_C, xdot_kite_D,xdot_kite_kcu,xdot_above_kite,...
    CL_spline_coefs, CD_spline_coefs, rho_air, A_Kite,K,g_vec, m_A, m_B, m_C, m_D, d0, c0,...
    ls_AC, ls_AB, ls_AKcu, ls_AD, ls_CB, ls_CD, ls_CKcu, ls_DKcu, ls_DB,l_s_BP, c_1_TR )

% Calculation of depower AoA and steering AoA
alpha_d = 0;(u_d - u_d_0)/(u_d_max - u_d_0) * alpha_d_max;
alpha_s = 0;(u_s - u_s_0)/(1+ K_d_s * (alpha_d /alpha_d_max) ) * alpha_s_max;

% Calculation of unity vectors of the kite body fixed frame
x_kite_Pc = 0.5 * (x_kite_C + x_kite_D);
e_z_k = (x_kite_Pc - x_kite_B)/sqrt((x_kite_Pc - x_kite_B)'*(x_kite_Pc - x_kite_B));
e_y_k = (x_kite_C - x_kite_D)/sqrt((x_kite_C - x_kite_D)'*(x_kite_C - x_kite_D));
e_x_k = [ e_y_k(2)*e_z_k(3) - e_y_k(3)*e_z_k(2);
    e_y_k(3)*e_z_k(1) - e_y_k(1)*e_z_k(3);
    e_y_k(1)*e_z_k(2) - e_y_k(2)*e_z_k(1)];

% Calculation of the apparent wind speeds at the 3 lifting surfaces
v_a_k_B = v_w_vec - xdot_kite_B;
v_a_k_C = v_w_vec - xdot_kite_C;
v_a_k_D = v_w_vec - xdot_kite_D;

% Calculation of the apparent wind speeds in xy and xz plane
v_a_B_xz = v_a_k_B - (v_a_k_B'*e_y_k)*e_y_k;
v_a_C_xy = v_a_k_C - (v_a_k_C'*e_z_k)*e_z_k;
v_a_D_xy = v_a_k_D - (v_a_k_D'*e_z_k)*e_z_k;

% Calculation of angles of attack
alpha_B  = pi - acos( (v_a_B_xz'*e_x_k)/sqrt(v_a_B_xz'*v_a_B_xz) ) - alpha_d + alpha_0;
alpha_C  = pi - acos( (v_a_C_xy'*e_x_k)/sqrt(v_a_C_xy'*v_a_C_xy) ) - alpha_s + alpha_s_0;
alpha_D  = pi - acos( (v_a_D_xy'*e_x_k)/sqrt(v_a_D_xy'*v_a_D_xy) ) + alpha_s + alpha_s_0;

% Calculation of Cl(alpha)_i and Cd(alpha)_i based on the spline
% coefficients
[ C_L_B, C_D_B ] = calcCLandCD_4pKite( alpha_B,CL_spline_coefs,CD_spline_coefs );
[ C_L_C, C_D_C ] = calcCLandCD_4pKite( alpha_C,CL_spline_coefs,CD_spline_coefs );
[ C_L_D, C_D_D ] = calcCLandCD_4pKite( alpha_D,CL_spline_coefs,CD_spline_coefs);

% Calculate the lift and drag forces of the lifting surfaces
[ F_L_B, F_L_C, F_L_D,...
    F_D_B, F_D_C, F_D_D  ] = calc4pKiteForces( C_L_B,C_L_C,C_L_D,...
    C_D_B, C_D_C, C_D_D,...
    rho_air, A_Kite, ASideRel,K,...
    e_y_k, e_z_k,...
    v_a_k_B, v_a_k_C, v_a_k_D, ...
    v_a_B_xz, v_a_C_xy, v_a_D_xy);

% Spring-Damper forces
% Constant bridle line (as defined in the setup_KiteModel_4points.m script)
% Notation: z.B. AC => x_A - x_C => belongs to forces of inertia

c = c0;
d = d0;

f_AC = calcSpringDamperForce_Bridle(c, norm(x_kite_A-x_kite_C) , ls_AC, d, x_kite_A - x_kite_C, xdot_kite_A - xdot_kite_C, 1 );
f_AB = calcSpringDamperForce_Bridle(c, norm(x_kite_A-x_kite_B) , ls_AB, d, x_kite_A - x_kite_B, xdot_kite_A - xdot_kite_B, 1 );
f_AD = calcSpringDamperForce_Bridle(c, norm(x_kite_A-x_kite_D) , ls_AD, d, x_kite_A - x_kite_D, xdot_kite_A - xdot_kite_D, 1 );
f_A_kcu = calcSpringDamperForce_Bridle(c, norm(x_kite_A-x_kite_kcu) , ls_AKcu, d, x_kite_A - x_kite_kcu, xdot_kite_A - xdot_kite_kcu, 1 );
f_CA = -f_AC;
f_CD = calcSpringDamperForce_Bridle(c, norm(x_kite_C-x_kite_D) , ls_CD, d, x_kite_C - x_kite_D, xdot_kite_C - xdot_kite_D, 1 );
f_CB = calcSpringDamperForce_Bridle(c, norm(x_kite_C-x_kite_B) , ls_CB, d, x_kite_C - x_kite_B, xdot_kite_C - xdot_kite_B, 1 );
f_C_kcu = calcSpringDamperForce_Bridle(c, norm(x_kite_C-x_kite_kcu) , ls_CKcu, d, x_kite_C - x_kite_kcu, xdot_kite_C - xdot_kite_kcu, 1 );
f_DA = -f_AD;
f_DC = -f_CD;
f_DB = calcSpringDamperForce_Bridle(c, norm(x_kite_D-x_kite_B) , ls_DB, d, x_kite_D - x_kite_B, xdot_kite_D - xdot_kite_B, 1 );
f_D_kcu = calcSpringDamperForce_Bridle(c, norm(x_kite_D-x_kite_kcu) , ls_DKcu, d, x_kite_D - x_kite_kcu, xdot_kite_D - xdot_kite_kcu, 1 );
f_BA = -f_AB;
f_BC = -f_CB;
f_BD = -f_DB;
f_above_kite = calcSpringDamperForce(c0, norm(x_above_kite-x_kite_B) , l_s_BP, d0, x_above_kite - x_kite_B, xdot_above_kite - xdot_kite_B, 1 );

x_kite_A_dotdot = 1/m_A*( - m_A*g_vec - f_AC - f_AB - f_A_kcu );
x_kite_B_dotdot = 1/m_B*(F_L_B + F_D_B - m_B*g_vec - f_BA - f_BC - f_BD + f_above_kite  );
x_kite_C_dotdot = 1/m_C*(F_L_C + F_D_C - m_C*g_vec - f_CA - f_CD - f_CB - f_C_kcu );
x_kite_D_dotdot = 1/m_D*(F_L_D + F_D_D - m_D*g_vec - f_DA - f_DC - f_DB - f_D_kcu );

x_dotdot_kite = [x_kite_A_dotdot;
    x_kite_B_dotdot;
    x_kite_C_dotdot;
    x_kite_D_dotdot];

v_a = norm( sign( v_a_k_B ) * max( abs( norm(v_a_k_B) ), 0.1) );
Psi_dot = c_1_TR * v_a * (u_s-u_s_0)/(1+K_d_s*(u_d - u_d_0)/(u_d_max - u_d_0)    ); % Turn rate law without gravity compensation (ref. equaion 6.11, Fechner)
end

== matlab function model_tmp_4p/Plant/Tether_Kite_Tether_UAV_Dynamics_4P/UAV_Model/Rotate thrust vector according to attitude ==
  data: u_Thrust_I input; eta input; u_Thrust_B output
function u_Thrust_B   = thrust_Bz_direction(  u_Thrust_I, eta) 

phi = eta(1); 
theta = eta(2); 
psi = eta(3); 

% Rotate thrust vector such that it is perpendicular to the "rotor blades"
u_Thrust_B = [cos(psi)*cos(theta), sin(psi)*cos(theta), -sin(theta); 
            cos(psi)*sin(theta)*sin(phi)-sin(psi)*cos(phi), sin(psi)*sin(theta)*sin(phi)+cos(psi)*cos(phi), cos(theta)*sin(phi); 
            cos(psi)*sin(theta)*cos(phi)+sin(psi)*sin(phi), sin(psi)*sin(theta)*cos(phi)-cos(psi)*sin(phi), cos(theta)*cos(phi)] *...
            [0;0;u_Thrust_I];

== matlab function model_tmp_4p/Controller/Outer_Loop_Position/Adaptive_Augmentation/Proj(Theta_hat, GammaY)_1column/Proj(Theta,Theta_dot) ==
  data: flag output; f input; gradf input; Theta_dot input; Theta_hat_dot_ output; direction output; orthogonal_part output
function  [flag,Theta_hat_dot_, direction, orthogonal_part] = fcn(f, gradf, Theta_dot )
%#codegen


if ( f > 0 && Theta_dot'*gradf > 0 )
    flag  = 1;
    direction = Theta_dot'*gradf;
    Theta_hat_dot_ = Theta_dot - f * ( (gradf*gradf') / (gradf'*gradf) * Theta_dot )   ;
    orthogonal_part = f * ( (gradf*gradf') / (gradf'*gradf) * Theta_dot );
else
    direction = Theta_dot'*gradf;
    flag = 0;
    Theta_hat_dot_ =  Theta_dot;
    orthogonal_part = zeros(3,1);
end

== matlab function model_tmp_4p/Controller/Outer_Loop_Position/Adaptive_Augmentation/Proj(Theta_hat, GammaY)_1column/calculate_f ==
  data: theta_hat input; f output; Theta_max input; epsilon input
function f   = fcn(theta_hat,Theta_max, epsilon )
%#codegen
f = ( (1+epsilon)*norm(theta_hat)^2 - (Theta_max)^2 ) / (epsilon*(Theta_max)^2);

== matlab function model_tmp_4p/Controller/Outer_Loop_Position/Adaptive_Augmentation/Proj(Theta_hat, GammaY)_1column/calculate_gradf ==
  data: theta_hat input; gradf output; Theta_max input; epsilon input
function gradf = fcn(theta_hat,Theta_max, epsilon )
%#codegen
gradf = ( 2*(1+epsilon) ) / (epsilon*(Theta_max)^2) * theta_hat ;

== matlab function model_tmp_4p/Controller/Reelout_Speed_Control/Activation_Function ==
  data: d input; safety_factor_vro output
function safety_factor_vro = fcn(d)
%#codegen
zero_cross = 0.5;
% Sigmoid like function. Converges against 1 if d > zero_cross
% and against -1 if d < zero_cross. It is used to ensure that the 
% current tether length cannot enter the "safety-ball" around the drone.
safety_factor_vro = 2*( 1 ./ ( 1 + exp(-5*( d - zero_cross ) ) ) - 0.5 ) ;

== matlab function model_tmp_4p/Analysis/Evaluate_Lyapunovfunction ==
  data: xi input; V output; P input; d_hat input; gamma_d input; e_pred input; P_pred input; d_real input
function V = fcn(xi, P, d_hat, gamma_d, e_pred, P_pred,d_real)
%#codegen
d_real = [5;5;5];
d_tilde = -d_hat - d_real;
V = 0.5 * xi' * P * xi + ...
    0.5 * e_pred * P_pred * e_pred' + ...
    0.5 * trace(d_tilde * 1 / gamma_d * d_tilde');

== matlab function model_tmp_4p/Plant/Tether_Kite_Tether_UAV_Dynamics_4P/Tethermodel_Kite2UAV/Tether_Kite2UAV ==
  data: launch_flag input; x_dotdot_p output; m_p parameter; g_vec parameter; xp_above input; xp input; xp_below input; xp_dot_above input; xp_dot input; xp_dot_below input; c0 parameter; d0 parameter; l_s_PUav parameter; l_s_BP parameter; CD_tether parameter; d_tether parameter; rho_air parameter; v_w_vec input
function x_dotdot_p   = fcn(launch_flag, m_p, g_vec, xp_above, xp, xp_below, xp_dot_above, xp_dot, xp_dot_below,...
                        c0, d0, l_s_PUav, l_s_BP, CD_tether, d_tether, rho_air, v_w_vec  )
%#codegen
% Tether forces from below and above
f_T_below = calcSpringDamperForce(c0, norm(xp - xp_below) , l_s_BP, d0, xp - xp_below, xp_dot - xp_dot_below, 1 );
f_T_above = calcSpringDamperForce(c0, norm(xp_above - xp), l_s_PUav, d0, xp_above - xp, xp_dot_above - xp_dot, 1 );

v_a_p = v_w_vec - 0.5 * ( xp_dot + xp_dot_above ) ; 
Dp = calcSegmentDrag( xp_above - xp  , v_a_p, rho_air, CD_tether, d_tether );

if launch_flag
    x_dotdot_p = 1/m_p * ( f_T_above - m_p*g_vec  + Dp ); % Particle dynamics
else
    x_dotdot_p = 1/m_p * ( -f_T_below + f_T_above - m_p*g_vec  + Dp );  %
end
